simulink model "S_torce3"  (Simulink 2.00)
settings: Solver=ode5  StartTime=0.0  StopTime=200  FixedStep=0.1  MaxStep=0.1  RelTol=1e-3  AbsTol=1e-6
values from neighbouring files (symbols this model uses):
  A1 = 2    [torce11.m]    (also in torcell.mat; waag11.mat)
  A12 = 0.1    [torce11.m]    (also in torcell.mat; waag11.mat)
  A2 = 2    [torce11.m]    (also in torcell.mat; waag11.mat)
  g = 9.8    [ident21.mat]    (also in torce11.m = 9.81; torcell.mat = 9.81; waag11.m = 9.81; waag11.mat = 9.81)
undefined symbols (not defined in the file or in its folder): delta, Tz
settings Model: SaveTime=off  SaveOutput=off  ConsistencyChecking=off

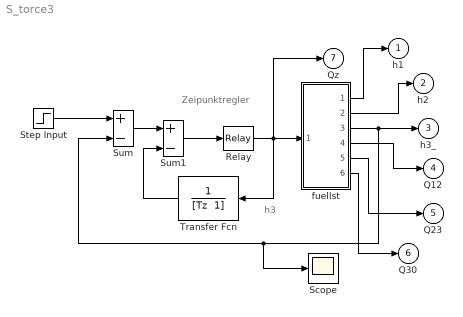
== system S_torce3 ==
  note: Zeipunktregler
  note: h3
  Relay : Relay  OnSwitchValue=delta  OffSwitchValue=-delta  OnOutputValue=Qz_rmax  OffOutputValue=Qz_rmin
  Scope : Scope
      settings: TickLabels=on  TimeRange=204.800000  YMin=-2.970000  YMax=2.970000  SaveToWorkspace=off  SaveName=ScopeData
  Step Input : Step  Time=1  Before=0  After=1
  Sum : Sum  Inputs=+-
  Sum1 : Sum  Inputs=+-
  Transfer Fcn : TransferFcn  Orientation=left  Numerator=[1 ]  Denominator="[Tz  1]"
  "fuellst " : Subsystem
  h1 : Outport  Port=1  InitialOutput=0
  h2 : Outport  Port=2  InitialOutput=0
  h3_ : Outport  Port=3  InitialOutput=0
  Q12 : Outport  Port=4  InitialOutput=0
  Q23 : Outport  Port=5  InitialOutput=0
  Q30 : Outport  Port=6  InitialOutput=0
  Qz : Outport  Port=7  InitialOutput=0
  wires:
  "fuellst "/1(out_1) -> h1/1
  "fuellst "/2(out_3) -> h2/1
  "fuellst "/4(out_2) -> Q12/1
  "fuellst "/5(out_4) -> Q23/1
  "fuellst "/6(out_6) -> Q30/1
  "fuellst "/3(out_5) -> Scope/1, Sum/2, h3_/1
  Step Input/1 -> Sum/1
  Relay/1 -> "fuellst "/1(in_1), Qz/1, Transfer Fcn/1
  Sum1/1 -> Relay/1
  Sum/1 -> Sum1/1
  Transfer Fcn/1 -> Sum1/2

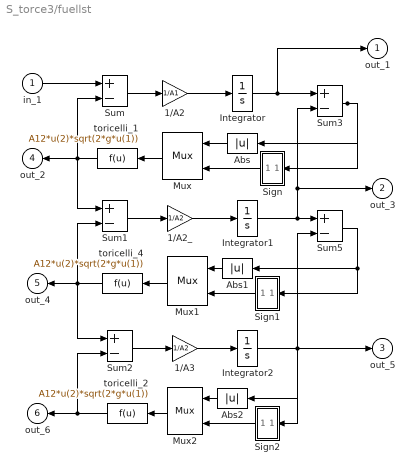
== system S_torce3/fuellst  ==
  in_1 : Inport  Port=1  PortWidth=-1  SampleTime=-1
  1/A2 : Gain  Gain=1/A1
  1/A2_ : Gain  Gain=1/A2
  1/A3 : Gain  Gain=1/A2
  Abs : Abs  Orientation=left
  Abs1 : Abs  Orientation=left
  Abs2 : Abs  Orientation=left
  Integrator : Integrator  ExternalReset=none  InitialConditionSource=internal  InitialCondition=0  LimitOutput=off  UpperSaturationLimit=inf  LowerSaturationLimit=-inf  ShowSaturationPort=off  ShowStatePort=off  AbsoluteTolerance=auto
  Integrator1 : Integrator  ExternalReset=none  InitialConditionSource=internal  InitialCondition=0  LimitOutput=off  UpperSaturationLimit=inf  LowerSaturationLimit=-inf  ShowSaturationPort=off  ShowStatePort=off  AbsoluteTolerance=auto
  Integrator2 : Integrator  ExternalReset=none  InitialConditionSource=internal  InitialCondition=0  LimitOutput=off  UpperSaturationLimit=inf  LowerSaturationLimit=-inf  ShowSaturationPort=off  ShowStatePort=off  AbsoluteTolerance=auto
  Mux : Mux  Orientation=left  Inputs=2
  Mux1 : Mux  Orientation=left  Inputs=2
  Mux2 : Mux  Orientation=left  Inputs=2
  Sign : Subsystem  Orientation=left
      mask Type: Sign
      mask Description: y = sign(x)
      mask Help: Sign Function:\n\t\t\ty = 1 if x > 0\n\t\t\ty = 0 if x = 0\n\t\t\ty = -1 if x < 0
      mask Display: plot(-50,-50,50,50,[-50,50],[0,0],[0,0],[-50,50],[-40,0],[-30,-30],[0,40],[30,30])
  Sign1 : Subsystem  Orientation=left
      mask Type: Sign
      mask Description: y = sign(x)
      mask Help: Sign Function:\n\t\t\ty = 1 if x > 0\n\t\t\ty = 0 if x = 0\n\t\t\ty = -1 if x < 0
      mask Display: plot(-50,-50,50,50,[-50,50],[0,0],[0,0],[-50,50],[-40,0],[-30,-30],[0,40],[30,30])
  Sign2 : Subsystem  Orientation=left
      mask Type: Sign
      mask Description: y = sign(x)
      mask Help: Sign Function:\n\t\t\ty = 1 if x > 0\n\t\t\ty = 0 if x = 0\n\t\t\ty = -1 if x < 0
      mask Display: plot(-50,-50,50,50,[-50,50],[0,0],[0,0],[-50,50],[-40,0],[-30,-30],[0,40],[30,30])
  Sum{,1..3,5} (5 alike) : Sum  Inputs=+-
  toricelli_1 : Fcn  Orientation=left  Expr=A12*u(2)*sqrt(2*g*u(1))
  toricelli_2 : Fcn  Orientation=left  Expr=A12*u(2)*sqrt(2*g*u(1))
  toricelli_4 : Fcn  Orientation=left  Expr=A12*u(2)*sqrt(2*g*u(1))
  out_1 : Outport  Port=1  InitialOutput=0
  out_3 : Outport  Port=2  InitialOutput=0
  out_5 : Outport  Port=3  InitialOutput=0
  out_2 : Outport  Orientation=left  Port=4  InitialOutput=0
  out_4 : Outport  Orientation=left  Port=5  InitialOutput=0
  out_6 : Outport  Orientation=left  Port=6  InitialOutput=0
  wires:
  Sum/1 -> 1/A2/1
  Sum1/1 -> 1/A2_/1
  Sum2/1 -> 1/A3/1
  1/A2/1 -> Integrator/1
  1/A2_/1 -> Integrator1/1
  1/A3/1 -> Integrator2/1
  Integrator1/1 -> Sum5/1, Sum3/2, out_3/1
  Integrator2/1 -> out_5/1, Sum5/2, Abs2/1, Sign2/1(in_1)
  toricelli_1/1 -> out_2/1, Sum/2, Sum1/1
  Sum3/1 -> Abs/1, Sign/1(in_1)
  Abs/1 -> Mux/1
  Mux/1 -> toricelli_1/1
  Sign/1(out_1) -> Mux/2
  Mux1/1 -> toricelli_4/1
  Sign1/1(out_1) -> Mux1/2
  Sum5/1 -> Sign1/1(in_1), Abs1/1
  Abs1/1 -> Mux1/1
  toricelli_4/1 -> out_4/1, Sum1/2, Sum2/1
  Abs2/1 -> Mux2/1
  Mux2/1 -> toricelli_2/1
  Sign2/1(out_1) -> Mux2/2
  toricelli_2/1 -> out_6/1, Sum2/2
  in_1/1 -> Sum/1
  Integrator/1 -> Sum3/1, out_1/1

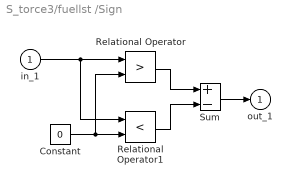
== system S_torce3/fuellst /Sign ==
  in_1 : Inport  Port=1  PortWidth=-1  SampleTime=-1
  Constant : Constant  Value=0
  Relational Operator : RelationalOperator  Operator=>
  Relational Operator1 : RelationalOperator  Operator=<
  Sum : Sum  Inputs=+-
  out_1 : Outport  Port=1  InitialOutput=0
  wires:
  Sum/1 -> out_1/1
  Relational Operator/1 -> Sum/1
  Relational Operator1/1 -> Sum/2
  Constant/1 -> Relational Operator1/2, Relational Operator/2
  in_1/1 -> Relational Operator/1, Relational Operator1/1

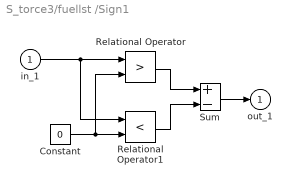
== system S_torce3/fuellst /Sign1 ==
  in_1 : Inport  Port=1  PortWidth=-1  SampleTime=-1
  Constant : Constant  Value=0
  Relational Operator : RelationalOperator  Operator=>
  Relational Operator1 : RelationalOperator  Operator=<
  Sum : Sum  Inputs=+-
  out_1 : Outport  Port=1  InitialOutput=0
  wires:
  Sum/1 -> out_1/1
  Relational Operator/1 -> Sum/1
  Relational Operator1/1 -> Sum/2
  Constant/1 -> Relational Operator1/2, Relational Operator/2
  in_1/1 -> Relational Operator/1, Relational Operator1/1

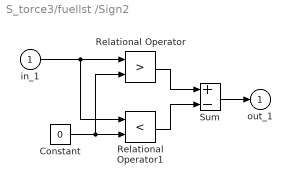
== system S_torce3/fuellst /Sign2 ==
  in_1 : Inport  Port=1  PortWidth=-1  SampleTime=-1
  Constant : Constant  Value=0
  Relational Operator : RelationalOperator  Operator=>
  Relational Operator1 : RelationalOperator  Operator=<
  Sum : Sum  Inputs=+-
  out_1 : Outport  Port=1  InitialOutput=0
  wires:
  Sum/1 -> out_1/1
  Relational Operator/1 -> Sum/1
  Relational Operator1/1 -> Sum/2
  Constant/1 -> Relational Operator1/2, Relational Operator/2
  in_1/1 -> Relational Operator/1, Relational Operator1/1
